simulink model "ultrasonic"  (R2023b)
settings: Solver=FixedStepDiscrete  StartTime=0.0  StopTime=10.0  FixedStep=0.01  RelTol=1e-3
libraries: simulink x2
settings Model: Creator=LENOVO-MCC  LastModifiedBy=LENOVO-MCC
settings OptimizationCC: DefaultParameterBehavior=Inlined  EnhancedBackFolding=on  PassReuseOutputArgsAs=Individual arguments  ZeroExternalMemoryAtStartup=off  ZeroInternalMemoryAtStartup=off  OptimizeBlockOrder=speed  DifferentSizesBufferReuse=on  OptimizationCustomize=off  EfficientTunableParamExpr=on
settings DebuggingCC: ParameterTunabilityLossMsg=error
settings SFSimCC: MATLABDynamicMemAlloc=off
settings RTWCC: Description=Embedded Coder  SystemTargetFile=ert.tlc  GenCodeOnly=on  TemplateMakefile=ert_default_tmf  GenerateReport=on  LaunchReport=on  GenerateCodeMetricsReport=on
settings CodeAppCC: ForceParamTrailComments=on  IgnoreCustomStorageClasses=off  OperatorAnnotations=on  SimulinkDataObjDesc=on  SFDataObjDesc=on  InsertBlockDesc=on
settings ERTTargetCC: TargetLangStandard=C99 (ISO)  GenerateSampleERTMain=on  InlinedParameterPlacement=NonHierarchical  ERTCustomFileTemplate=example_file_process.tlc

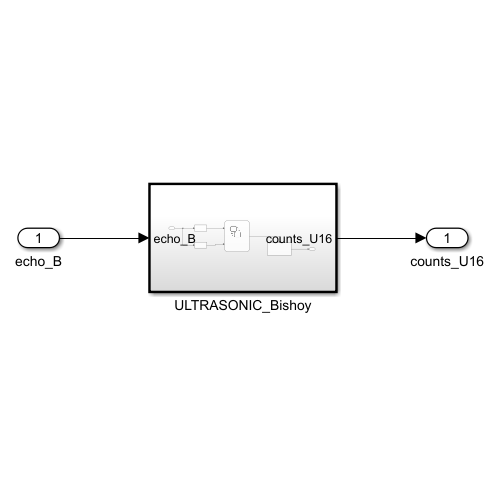
[thumbnail: Simulink's stored preview of the top-level diagram]
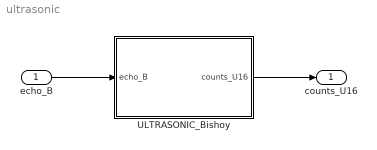
== system ultrasonic ==
  echo_B : Inport  OutDataTypeStr=boolean
  ULTRASONIC_Bishoy : Subsystem  TreatAsAtomicUnit=on
      settings: RTWFcnNameOpts=Use subsystem name  RTWFileNameOpts=Use subsystem name
  counts_U16 : Outport
  wires:
  echo_B/1 -> ULTRASONIC_Bishoy/1(echo_B)
  ULTRASONIC_Bishoy/1(counts_U16) -> counts_U16/1

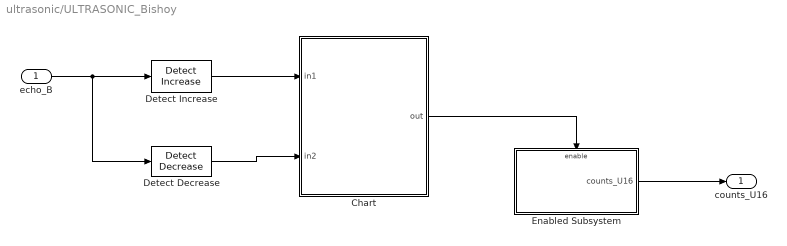
== system ultrasonic/ULTRASONIC_Bishoy ==
  echo_B : Inport  OutDataTypeStr=boolean
  Chart : Stateflow chart  TreatAsAtomicUnit=on
  Detect Decrease : simulink/Logic and Bit Operations/Detect Decrease  vinit=0.0  OutDataTypeStr=boolean
      settings: LibrarySourceBlock=|
      | hdlsllib/Logic and Bit
      | Operations/Detect
      | Decrease
  Detect Increase : simulink/Logic and Bit Operations/Detect Increase  vinit=0.0  OutDataTypeStr=boolean
  Enabled Subsystem : Subsystem  TreatAsAtomicUnit=on
  counts_U16 : Outport
  wires:
  echo_B/1 -> Detect Decrease/1, Detect Increase/1
  Detect Increase/1 -> Chart/1(in1)
  Detect Decrease/1 -> Chart/2(in2)
  Chart/1(out) -> Enabled Subsystem/Enable
  Enabled Subsystem/1(counts_U16) -> counts_U16/1

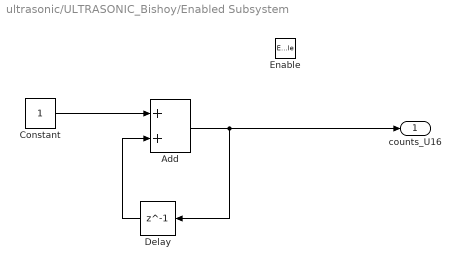
== system ultrasonic/ULTRASONIC_Bishoy/Enabled Subsystem ==
  Enable : EnablePort  StatesWhenEnabling=reset
  Add : Sum
  Constant : Constant
  Delay : Delay  DelayLength=1
  counts_U16 : Outport
  wires:
  Constant/1 -> Add/1
  Add/1 -> counts_U16/1, Delay/1
  Delay/1 -> Add/2

== stateflow chart ultrasonic/ULTRASONIC_Bishoy/Chart ==
  state hold
    en:
    out=false;
  state change
    en:
    out=true;
  (default) -> hold
  hold -> change : [in1 == true]
  change -> hold : [in2 == true]
  data: in1 input; in2 input; out output
